simulink model "analog_adapt2"  (Simulink 10.2)
settings: Solver=VariableStepAuto  StartTime=0.0  StopTime=20  RelTol=1e-3
libraries: dsparch4 x1, simulink x1, dspadpt3 x1
settings Model: Creator=shiva  LastModifiedBy=shiva
settings DataIOCC: SaveFormat=Dataset  SignalLoggingSaveFormat=Dataset  ReturnWorkspaceOutputs=on
settings OptimizationCC: LifeSpan=auto
settings DebuggingCC: UnderspecifiedInitializationDetection=Simplified  MergeDetectMultiDrivingBlocksExec=error  FcnCallInpInsideContextMsg=error  SFUnexpectedBacktrackingDiag=error  SFNoUnconditionalDefaultTransitionDiag=error  SFExecutionAtInitializationDiag=warning  ArithmeticOperatorsInVariantConditions=error
settings HardwareCC: ProdBitPerPointer=64  ProdBitPerSizeT=64  ProdBitPerPtrDiffT=64  ProdLargestAtomicFloat=Float  ProdIntDivRoundTo=Zero  ProdEndianess=LittleEndian  ProdWordSize=64  ProdHWDeviceType=Intel->x86-64 (Windows64)
settings ModelReferenceCC: PropagateSignalLabelsOutOfModel=on
settings SFSimCC: SimUseLocalCustomCode=on  CustomCodeUndefinedFunction=FilterOut
settings RTWCC: RTWUseLocalCustomCode=on
settings CodeAppCC: StateflowObjectComments=off
settings GRTTargetCC: TargetLangStandard=C99 (ISO)  CombineOutputUpdateFcns=on  GRTInterface=off
settings ConfigComp: CovMetricSettings=dwe  CovSaveCumulativeToWorkspaceVar=off  CovSaveSingleToWorkspaceVar=off  CovExternalEMLEnable=on

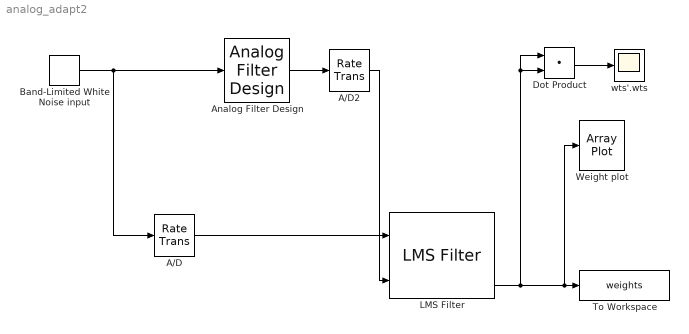
== system analog_adapt2 ==
  A/D : RateTransition  OutPortSampleTime=125*10^-6
  A/D2 : RateTransition  OutPortSampleTime=125*10^-6
  Analog Filter Design : dsparch4/Analog Filter Design  method=Butterworth  filttype=Lowpass  N=8  Wlo=12560  Whi=80  Rp=2  Rs=40
  Band-Limited White Noise input : simulink/Sources/Band-Limited White Noise  Cov=[1]  Ts=125*10^-6  seed=[23341]
  Dot Product : DotProduct  InputSameDT=on  OutDataTypeStr=Inherit: Inherit via internal rule
  LMS Filter : dspadpt3/LMS Filter  Algo=Normalized LMS  L=99  stepflag=Dialog  mu=0.01  leakage=1  ic=0  Adapt=off  resetflag=None  weights=on  addnparflag=off  roundingMode=Floor  overflowMode=off
      settings: SourceProductBaseCode=DS
  To Workspace : ToWorkspace  VariableName=weights  SampleTime=-1
      settings: MaxDataPoints=99  Save2DSignal=2-D array (concatenate along first dimension)
  Weight plot : ArrayPlot
  wts'.wts : Scope
  wires:
  Band-Limited White Noise input/1 -> A/D/1, Analog Filter Design/1
  Analog Filter Design/1 -> A/D2/1
  A/D2/1 -> LMS Filter/2
  A/D/1 -> LMS Filter/1
  LMS Filter/3 -> Dot Product/1, Dot Product/2, Weight plot/1, To Workspace/1
  Dot Product/1 -> wts'.wts/1
